simulink model "transf2"  (Simulink 5.0)
settings: Solver=ode45  StartTime=0.0  StopTime=100  RelTol=1e-3
undefined symbols (not defined in the file): sigbuilder_block
settings Model: Creator=cousot  LastModifiedBy=cousot  ExtModeAutoUpdateStatusClock=off

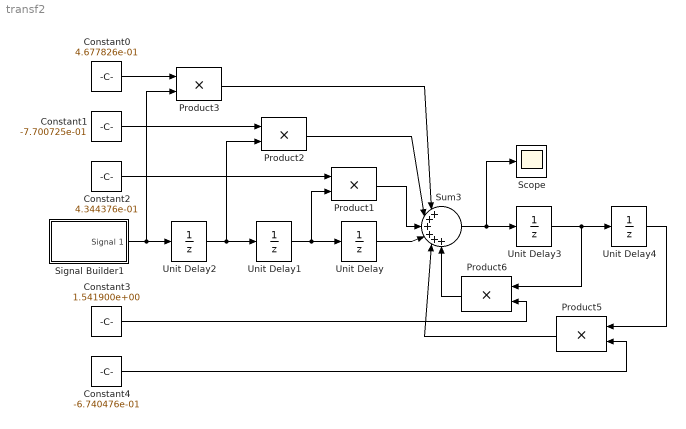
== system transf2 ==
  Constant0 : Constant  Value=4.677826e-01
  Constant1 : Constant  Value=-7.700725e-01
  Constant2 : Constant  Value=4.344376e-01
  Constant3 : Constant  Value=1.541900e+00
  Constant4 : Constant  Value=-6.740476e-01
  Product1 : Product  SaturateOnIntegerOverflow=on
  Product2 : Product  SaturateOnIntegerOverflow=on
  Product3 : Product  SaturateOnIntegerOverflow=on
  Product5 : Product  Orientation=left  SaturateOnIntegerOverflow=on
  Product6 : Product  Orientation=left  SaturateOnIntegerOverflow=on
  Scope : Scope
      settings: TimeRange=100
  Signal Builder1 : Subsystem  Tag=STV Subsys  LoadFcn=sigbuilder_block('open',[281.298 229.455 574.116 415.706 ]);  StartFcn=sigbuilder_block('start');  StopFcn=sigbuilder_block('stop');  ClipboardFcn=sigbuilder_block('clipboard');  mask(Sigbuilder block){}
      mask help: Sigbuilder GUI
      mask init:
      | if ~strcmp(get_param(bdroot(gcb),'SimulationStatus'),'stopped') tuvar = sigbuilder_block('maskInit'); end
      settings: CopyFcn=sigbuilder_block('copy');  DeleteFcn=sigbuilder_block('delete');  ModelCloseFcn=sigbuilder_block('modelClose');  PreSaveFcn=sigbuilder_block('preSave');  NameChangeFcn=sigbuilder_block('namechange');  OpenFcn=sigbuilder_block('open',[127.688 64.3241 665.322 389.785 ]);  CloseFcn=sigbuilder_block('close');
      mask Display: plot(0,0,100,100,[10,10,40,40,10],[80,20,20,80,80],[40,10],[50,50], [40,27,10],[65,72,56],[40,25,25,10],[28,28,43,43]);
  Sum3 : Sum  Inputs=|++++++  SaturateOnIntegerOverflow=on
  Unit Delay{,1..4} (5 alike) : UnitDelay
  wires:
  Unit Delay/1 -> Sum3/4
  Unit Delay1/1 -> Product1/2, Unit Delay/1
  Unit Delay2/1 -> Unit Delay1/1, Product2/2
  Signal Builder1/1(Signal 1) -> Product3/2, Unit Delay2/1
  Constant0/1 -> Product3/1
  Constant2/1 -> Product1/1
  Product3/1 -> Sum3/1
  Product2/1 -> Sum3/2
  Product1/1 -> Sum3/3
  Sum3/1 -> Unit Delay3/1, Scope/1
  Unit Delay3/1 -> Unit Delay4/1, Product6/1
  Constant1/1 -> Product2/1
  Product5/1 -> Sum3/5
  Product6/1 -> Sum3/6
  Unit Delay4/1 -> Product5/1
  Constant3/1 -> Product6/2
  Constant4/1 -> Product5/2

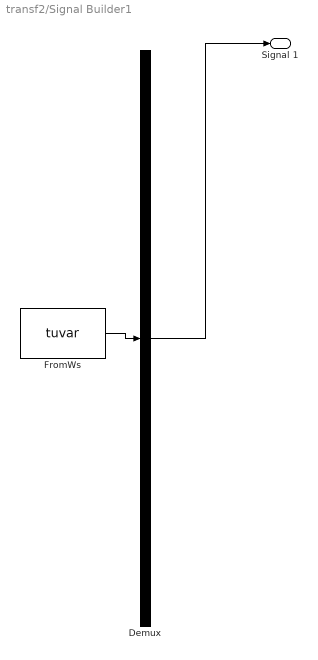
== system transf2/Signal Builder1 ==
  Demux : Demux  Tag=STV Demux  Outputs=1
  FromWs : FromWorkspace  Tag=STV FromWs  VariableName=tuvar  SampleTime=0  SigBuilderData=DataTag0
  Signal 1 : Outport  Tag=STV Outport
  wires:
  Demux/1 -> Signal 1/1
  FromWs/1 -> Demux/1
